simulink model "moter_1"  (R2018a)
settings: Solver=VariableStepAuto  StartTime=0.0  StopTime=2  RelTol=1e-8
settings Model: Creator=Abarhand  LastModifiedBy=Abarhand

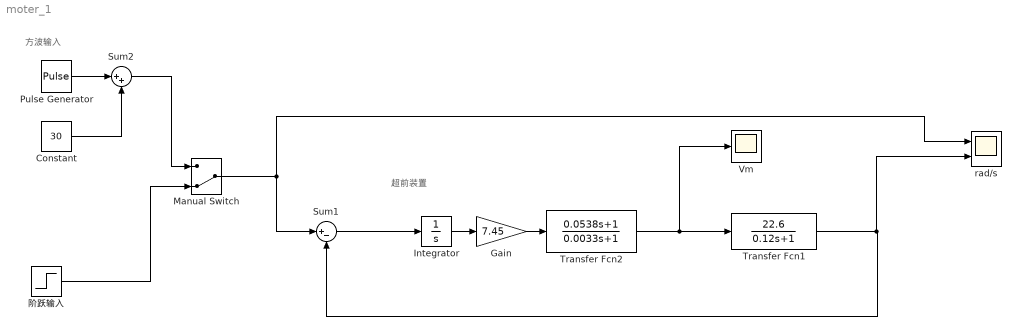
== system moter_1 ==
  note: 方波输入
  note: 超前装置
  Constant : Constant  Value=30
  Gain : Gain  Gain=7.45
  Integrator : Integrator
  Manual Switch : ManualSwitch  CurrentSetting=0
  Pulse Generator : DiscretePulseGenerator  PulseType=Time based  Amplitude=10  Period=5  PulseWidth=50
  Sum1 : Sum  Inputs=|+-
  Sum2 : Sum  Inputs=|++
  Transfer Fcn1 : TransferFcn  Numerator=[22.6]  Denominator=[0.12 1 ]
  Transfer Fcn2 : TransferFcn  Numerator=[0.0538 1]  Denominator=[0.0033 1]
  Vm : Scope
  rad/s : Scope  NumInputPorts=2
      settings: Tag=rad/s
  阶跃输入 : Step  SampleTime=0
  wires:
  Sum2/1 -> Manual Switch/1
  Gain/1 -> Transfer Fcn2/1
  Integrator/1 -> Gain/1
  Sum1/1 -> Integrator/1
  Transfer Fcn1/1 -> rad/s/2, Sum1/2
  Transfer Fcn2/1 -> Vm/1, Transfer Fcn1/1
  Pulse Generator/1 -> Sum2/1
  Constant/1 -> Sum2/2
  阶跃输入/1 -> Manual Switch/2
  Manual Switch/1 -> Sum1/1, rad/s/1
